simulink model "P8"  (R2015a)
settings: Solver=ode45  StartTime=0.0  StopTime=10.0  RelTol=1e-3
settings Model: Creator=joao  LastModifiedBy=Diogo
settings DataIOCC: SignalLoggingSaveFormat=ModelDataLogs
settings OptimizationCC: ExpressionDepthLimit=2147483647
settings DebuggingCC: UnderspecifiedInitializationDetection=Classic  MergeDetectMultiDrivingBlocksExec=none  SolverPrmCheckMsg=warning  FcnCallInpInsideContextMsg=EnableAllAsWarning  StateNameClashWarn=warning
settings GRTTargetCC: CombineOutputUpdateFcns=off  GRTInterface=on

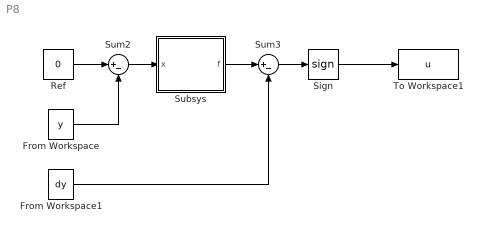
== system P8 ==
  From Workspace : FromWorkspace  VariableName=y
  From Workspace1 : FromWorkspace  VariableName=dy
  Ref : Constant  Value=0  VectorParams1D=off
  Sign : Signum
  "Subsys " : Subsystem
  Sum2 : Sum  Inputs=|+-
  Sum3 : Sum  Inputs=|+-
  To Workspace1 : ToWorkspace  VariableName=u  SampleTime=-1
  wires:
  Ref/1 -> Sum2/1
  Sum2/1 -> "Subsys "/1(x)
  Sum3/1 -> Sign/1
  Sign/1 -> To Workspace1/1
  From Workspace/1 -> Sum2/2
  From Workspace1/1 -> Sum3/2
  "Subsys "/1("f ") -> Sum3/1

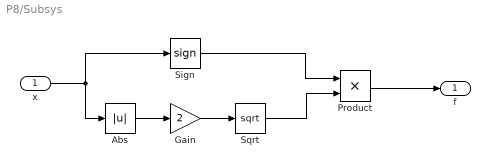
== system P8/Subsys  ==
  x : Inport
  Abs : Abs
  Gain : Gain  Gain=2
  Product : Product
  Sign : Signum
  Sqrt : Sqrt  SaturateOnIntegerOverflow=on
  "f " : Outport
  wires:
  Abs/1 -> Gain/1
  Gain/1 -> Sqrt/1
  Sqrt/1 -> Product/2
  Product/1 -> "f "/1
  Sign/1 -> Product/1
  x/1 -> Sign/1, Abs/1
